simulink model "EstudioVirtual"  (Simulink 7.9)
settings: Solver=ode3  SolverMode=SingleTasking  StartTime=0.0  StopTime=10.0  RelTol=1e-3
PreLoadFcn:
  | waijung.modelPreload; % Required for working with Waijung Blockset. Do not remove.
undefined symbols (not defined in the file or in its folder): ARM, Link, LQFP100, MDK, ST, STM32F407VG, STM32F4DISCOVERY
libraries: stm32f4_io_lib x4, stm32f4_device_config_lib x1
CloseFcn:
  | waijung.modelClose; % Required for working with Waijung Blockset. Do not remove.
settings Model: Creator=Lithium  LastModifiedBy=Lithium
settings OptimizationCC: OptimizeModelRefInitCode=on  LifeSpan=1
settings HardwareCC: ProdEndianess=LittleEndian  ProdHWDeviceType=ARM Compatible->Cortex - M4  TargetEndianess=LittleEndian  TargetHWDeviceType=ARM Compatible->Cortex - M4
settings RTWCC: SystemTargetFile=stm32f4.tlc  GenerateMakefile=off  TemplateMakefile=ert_default_tmf  Description=STM32F4 Target  ProcessScript=stm32f4_make_rtw_hook
settings CodeAppCC: IgnoreCustomStorageClasses=off
settings STFCustomTargetCC: CodeReplacementLibrary=ANSI_C  ModelReferenceCompliant=off  CombineOutputUpdateFcns=on  ERTCustomFileBanners=on  SupportContinuousTime=off  SupportNonInlinedSFcns=off  GRTInterface=off  SystemTargetFile=stm32f4.tlc
settings ERTTargetCC: CodeReplacementLibrary=ANSI_C  MultiwordLength=2048  ModelReferenceCompliant=off  ParMdlRefBuildCompliant=off  CompOptLevelCompliant=off  ConcurrentExecutionCompliant=off  ERTFirstTimeCompliant=off  ModelStepFunctionPrototypeControlCompliant=off  CPPClassGenCompliant=off  InlinedParameterPlacement=NonHierarchical  ERTSrcFileBannerTemplate=stm32f4_code_template.cgt  ERTHdrFileBannerTemplate=stm32f4_code_template.cgt  ERTDataSrcFileTemplate=stm32f4_code_template.cgt  ERTDataHdrFileTemplate=stm32f4_code_template.cgt  ERTCustomFileTemplate=stm32f4_file_process.tlc  ConvertIfToSwitch=off  SuppressUnreachableDefaultCases=off

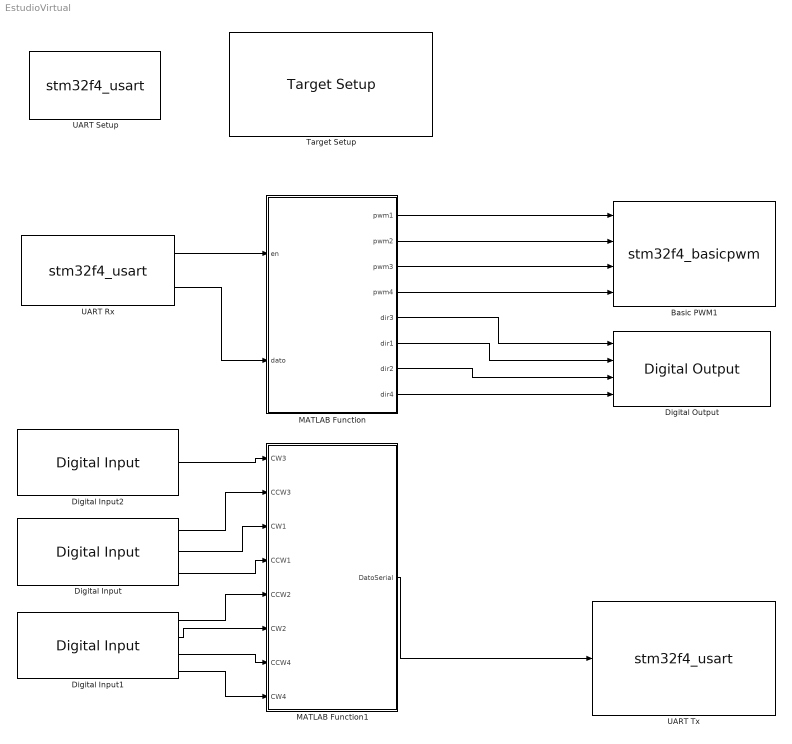
== system EstudioVirtual ==
  Basic PWM1 : S-Function  FunctionName=stm32f4_basicpwm  Parameters=timer,pwmperiod,ch1pin,ch2pin,ch3pin,ch4pin,sampletime,sampletimestr,blockid,apb,portstr,pinstr,pinmat,timarr,timprescale,chmat,polaritystr  EnableBusSupport=off  mask(stm32f4_basicpwm){timer=1, pwmperiod=0.0001, polarity=Active High, polaritystr=TIM_OCPolarity_High, ch1pin=E9, ch2pin=E11, ch3pin=E13, ch4pin=E14, sampletime=0.01, sampletimestr=-1, blockid=BasicPWM1, portpinstr=E9,E11,E13,E14, enablecustomportlabel=on, cinputportlabel=PWM1, PWM2, PWM3, PWM4, coutputportlabel=0, apb=2, portstr=["E"], pinstr=["GPIO_Pin_9 | GPIO_Pin_11 | GPIO_Pin_13 | GPIO_Pin_14"], pinmat=[4 9 11 13 14], timarr=16799, timprescale=0, chmat=[1  2  3  4]}
      mask prompts: pwmperiod "PWM Period (seconds)"; ch1pin "Channel 1"; ch2pin "Channel 2"; ch3pin "Channel 3"; ch4pin "Channel 4"; sampletime "Sample time (sec)"; sampletimestr "Compiled sample time (sec) in string"; portpinstr "Port pin string"; enablecustomportlabel "Enable custom port labels"; cinputportlabel "Custom input port labels (Ex. In1, In2, In3)"; coutputportlabel "Custom output port labels (Ex. Out1, Out2, Out3)"; portstr "Port string"; pinstr "Pin string"; pinmat "Pin matrix"; timarr "Timer ARR"; timprescale "Timer PRESCALE"; chmat "Channel order"
      mask help:
      | This block implements basic Edge-aligned Pulse Width Modulation (PWM) generation.
      | All timers are 16-bit. The PWM period is fixed (per timer).
      mask init:
      | stm32f4_basicpwm_callback('init');
      mask Help: web(fullfile(waijungdocroot,'stm32f4_basicpwm.htm'),'-browser')
      mask StyleString: popup(1|2|3|4|5|8|9|10|11|12|13|14),edit,popup(Active High|Active Low),edit,popup(Not available - Do not use|E9|A8),popup(Not available - Do not use|E11|A9),popup(Not available - Do not use|E13|A10),popup(Not available - Do not use|E14|A11),edit,edit,edit,edit,checkbox,edit,edit,edit,edit,edit,edit,edit,edit,edit
      mask CallbackString: stm32f4_basicpwm_callback('timer');|stm32f4_basicpwm_callback('pwmperiod');|stm32f4_basicpwm_callback('polarity');||stm32f4_basicpwm_callback('ch1pin');|stm32f4_basicpwm_callback('ch2pin');|stm32f4_basicpwm_callback('ch3pin');|stm32f4_basicpwm_callback('ch4pin');|stm32f4_basicpwm_callback('sampletime');|stm32f4_basicpwm_callback('sampletimestr');|stm32f4_basicpwm_callback('blockid');||stm32f4_basicpwm_callback('enablecustomportlabel');|||||||||
      mask Display: text(0.95, 0.5, 'Timer: 1\nPolarity: Active High\nPeriod (sec) 0.0001\nTs (sec): -1','ver','middle','hor','right');port_label('input', 1,'PWM1 (E9)');port_label('input', 2,'PWM2 (E11)');port_label('input', 3,'PWM3 (E13)');port_label('input', 4,'PWM4 (E14)')
  Digital Input : stm32f4_io_lib/Digital Input  port=B  speed=100  porttype=Pull Up  porttypestr=UP  use_pin0=off  use_pin1=off  use_pin2=off  use_pin3=on  use_pin4=off  use_pin5=off  use_pin6=off  use_pin7=off  use_pin8=off  use_pin9=off  use_pin10=off  use_pin11=off  use_pin12=off  use_pin13=on  use_pin14=on  use_pin15=off  pinstr=GPIO_Pin_3 | GPIO_Pin_13 | GPIO_Pin_14  usedpinarray="[0  0  0  1  0  0  0  0  0  0  0  0  0  1  1  0]"  bitbandingstr=|  sampletime=0.01  sampletimestr=-1  blockid=DigitalInput  enablecustomportlabel=on  glabalinit=off  cinputportlabel=In1, In2  coutputportlabel=CCW3, CW1, CCW1
      | #define DigitalInput_B3 Peripheral_BB(GPIOB->IDR, 3)  /* Output pin */
      | #define DigitalInput_B13 Peripheral_BB(GPIOB->IDR, 13)  /* Output pin */
      | #define DigitalInput_B14 Peripheral_BB(GPIOB->IDR, 14)  /* Output pin */
  Digital Input1 : stm32f4_io_lib/Digital Input  port=E  speed=100  porttype=Pull Up  porttypestr=UP  use_pin0=off  use_pin1=off  use_pin2=off  use_pin3=off  use_pin4=off  use_pin5=on  use_pin6=on  use_pin7=on  use_pin8=off  use_pin9=off  use_pin10=off  use_pin11=off  use_pin12=on  use_pin13=off  use_pin14=off  use_pin15=off  pinstr=GPIO_Pin_5 | GPIO_Pin_6 | GPIO_Pin_7 | GPIO_Pin_12  usedpinarray="[0  0  0  0  0  1  1  1  0  0  0  0  1  0  0  0]"  bitbandingstr=|  sampletime=0.01  sampletimestr=-1  blockid=DigitalInput1  enablecustomportlabel=on  glabalinit=off  cinputportlabel=In1, In2  coutputportlabel=CCW2, CW2, CCW4, CW4
      | #define DigitalInput1_E5 Peripheral_BB(GPIOE->IDR, 5)  /* Output pin */
      | #define DigitalInput1_E6 Peripheral_BB(GPIOE->IDR, 6)  /* Output pin */
      | #define DigitalInput1_E7 Peripheral_BB(GPIOE->IDR, 7)  /* Output pin */
      | #define DigitalInput1_E12 Peripheral_BB(GPIOE->IDR, 12)  /* Output pin */
  Digital Input2 : stm32f4_io_lib/Digital Input  port=D  speed=100  porttype=Pull Up  porttypestr=UP  use_pin0=off  use_pin1=off  use_pin2=off  use_pin3=off  use_pin4=off  use_pin5=off  use_pin6=off  use_pin7=off  use_pin8=off  use_pin9=off  use_pin10=off  use_pin11=on  use_pin12=off  use_pin13=off  use_pin14=off  use_pin15=off  pinstr=GPIO_Pin_11  usedpinarray="[0  0  0  0  0  0  0  0  0  0  0  1  0  0  0  0]"  bitbandingstr="#define DigitalInput2_D11 Peripheral_BB(GPIOD->IDR, 11)  /* Output pin */"  sampletime=0.01  sampletimestr=-1  blockid=DigitalInput2  enablecustomportlabel=on  glabalinit=off  cinputportlabel=In1, In2  coutputportlabel=CW3
  Digital Output : stm32f4_io_lib/Digital Output  use_bitband=on  port=B  speed=100  porttype=Push Pull  porttypestr=PP  use_pin0=off  use_pin1=off  use_pin2=off  use_pin3=off  use_pin4=on  use_pin5=off  use_pin6=off  use_pin7=on  use_pin8=on  use_pin9=on  use_pin10=off  use_pin11=off  use_pin12=off  use_pin13=off  use_pin14=off  use_pin15=off  pinstr=GPIO_Pin_4 | GPIO_Pin_7 | GPIO_Pin_8 | GPIO_Pin_9  usedpinarray="[0  0  0  0  1  0  0  1  1  1  0  0  0  0  0  0]"  bitbandingstr=|  sampletime=-1  sampletimestr=-1  blockid=DigitalOutput  enablecustomportlabel=on  globalinit=off  cinputportlabel=Dir3, Dir1, Dir2, Dir4  coutputportlabel=0
      | #define DigitalOutput_B4 Peripheral_BB(GPIOB->ODR, 4)  /* Output pin */
      | #define DigitalOutput_B7 Peripheral_BB(GPIOB->ODR, 7)  /* Output pin */
      | #define DigitalOutput_B8 Peripheral_BB(GPIOB->ODR, 8)  /* Output pin */
      | #define DigitalOutput_B9 Peripheral_BB(GPIOB->ODR, 9)  /* Output pin */
  MATLAB Function : MATLAB Function  TreatAsAtomicUnit=on
  MATLAB Function1 : MATLAB Function  TreatAsAtomicUnit=on
  Target Setup : stm32f4_device_config_lib/Target Setup  Priority=100  compiler=MDK-ARM  previous_compiler=MDK-ARM  mcu=STM32F407VG (LQFP100); STM32F4DISCOVERY  mcustr=STM32F407VG  clockconfig=STM32F4DISCOVERY Default (HSEOSC-8MHz/HCLK-168MHz)  system_stm32f4xx_c_path=C:\Users\Lithium\Downloads\waijung14_12a\targets\stm32f4_target\stm32f4\utils\STM32F4xx_AN3988_V1.0.1\stm32f4_default\hseosc8mhz  showmemoryconfiguration=off  stacksize=0x2000  heapsize=0x2000  enableautocompiledownload=on  fullchiperase=off  programmerinterface=ST-Link  editctrlstr=on  compilercontrolstr=-c --cpu Cortex-M4.fp -g -O3 --apcs=interwork --split_sections $(INCLUDES)  assemblercontrolstr="--cpu Cortex-M4.fp -g --apcs=interwork  --xref $(INCLUDES)"  linkercontrolstr="--cpu Cortex-M4.fp --strict --scatter \"$(MODELNAME).sct\" --summary_stderr --info summarysizes --map --xref --callgraph --symbols --info sizes --info totals --info unused --info veneers  --list \".\\$(MODELNAME).map\" -o $(MODELNAME).axf"  runafterdownload=on  execprofile=None  profileruart=3  profilerbaud=500000  profilertxpin=D8  profilerinitstr=0.01,168000000,1680000,500000,0  manualsetsampletime=off  sampletime=0.01  blockid=TargetSetup  systickreloadvalue=1680000  hseval=8000000  lastprofileruart=3  hclk=168000000  flashorigin=0x08000000  flashlength=0x00100000  ramorigin=0x20000000  ramlength=0x00020000  useextram=off
  UART Rx : S-Function  Priority=1  FunctionName=stm32f4_usart  Parameters=configuration,uartmodule,transfer,baudrate,inputtype,outputtype,confstr,binheaderarray,binterminatorarray,asciiheader,asciiterminator,bindatalength,packetmode,varname,sampletime,sampletimestr,blockid  EnableBusSupport=off  mask(stm32f4_usart){configuration=Rx, uartmodule=6, baudrate=115200, databits=8, parity=No, stopbit=1, remaptxpin=Not used, remaprxpin=Not used, flowcontrol=None, remapctspin=Not used, remaprtspin=Not used, advanceoptions=off, rxbuffersize=512, txbuffersize=512, transfer=Non-Blocking, packetmode=Binary Vector, binheader='S', binterminator='0E', porttype_double=0, porttype_single=0, porttype_int8=3, porttype_uint8=0, porttype_int16=0, porttype_uint16=0, porttype_int32=0, porttype_uint32=0, asciiformat='value=%d,%f', rx_asciiterminator=CRLF (0x0D 0x0A - "\\r\\n"), tx_asciiterminator=LF (0x0A - "\\n"), storagename=<empty>, varname=, inputtype=[0], outputtype=[2 3  770], binheaderarray=[2 126  126], binterminatorarray=[1 14], bindatalength=3, asciiheader='value=%d,%f\\r\\n', asciiterminator=[2 13 10], sampletime=-1, sampletimestr=-1, blockid=UARTRx, confstr=[ "dummy", "0", "*", "*", "0", "*", "*", "0", "*", "*", "0", "*", "*", "2", "5", "6", "2", "5", "1", "512", "512", "2", "6", "115200", "8", "No", "1", "None", "USART6"], lastmodule=1}
      mask prompts: uartmodule "UART Module"; baudrate "Baud rate (bps)"; databits "Data bits"; stopbit "Stop bit"; remaptxpin "Tx Pin"; remaprxpin "Rx Pin"; flowcontrol "Hardware flow control"; remapctspin "HW Flow control, CTS Pin"; remaprtspin "HW Flow control, RTS Pin"; advanceoptions "Advance options"; rxbuffersize "Rx buffer size (bytes)"; txbuffersize "Tx buffer size (bytes)"; packetmode "Packet mode"; binheader "Binary header (example: '7E 7E')"; binterminator "Binary terminator (example: '03 03')"; porttype_double "Number of data port, type DOUBLE"; porttype_single "Number of data port, type SINGLE"; porttype_int8 "Number of data port, type INT8"; porttype_uint8 "Number of data port, type UINT8"; porttype_int16 "Number of data port, type INT16"; porttype_uint16 "Number of data port, type UINT16"; porttype_int32 "Number of data port, type INT32"; porttype_uint32 "Number of data port, type UINT32"; asciiformat "Ascii format"; rx_asciiterminator "End of packet"; tx_asciiterminator "End of packet"; storagename "Buffer"; varname "Var name"; inputtype "Input data type"; outputtype "Output data type"; binheaderarray "Binary header"; binterminatorarray "Binary terminator"; bindatalength "Binary data length"; asciiheader "Ascii header (printf format)"; asciiterminator "Ascii terminator"; sampletime "Sample time (sec)"; sampletimestr "Compiled sample time (sec) in string"; confstr "Configuration string"; lastmodule "Last module selected"
      mask help:
      | Data type for Ascii format
      | %u, %i, %d, %o, %x: uint32
      | %e, %g, %f: single
      | %c: int8
      mask init:
      | stm32f4_usart_callback('init');
      mask Help: web(fullfile(waijungdocroot,'stm32f4_usart_rx.htm'), '-browser')
      mask StyleString: popup(Setup|Tx|Rx),popup(1|2|3|4|5|6),edit,popup(8),popup(No|Odd|Even),popup(0.5|1|1.5|2),popup(Not used|A9|B6),popup(Not used|A10|B7),popup(None|RTS|CTS|RTS/CTS),popup(Not used|A11),popup(Not used|A12),checkbox,popup(16|32|64|128|256|512|1024|2048),popup(16|32|64|128|256|512|1024|2048),popup(Blocking|Non-Blocking),popup(Ascii|Binary|Binary Vector|String Buffer),edit,edit,edit,edit,edit,edit,edit,edit,edit,edit,edit,popup(CR (0x0D - "\\\\r")|LF (0x0A - "\\\\n")|CRLF (0x0D 0x0A - "\\\\r\\\\n")),popup(CR (0x0D - "\\\\r")|LF (0x0A - "\\\\n")|CRLF (0x0D 0x0A - "\\\\r\\\\n")|None),popup(<empty>),edit,edit,edit,edit,edit,edit,edit,edit,edit,edit,edit,edit,edit
      mask CallbackString: stm32f4_usart_callback('configuration');|stm32f4_usart_callback('uartmodule');|stm32f4_usart_callback('baudrate');||||||stm32f4_usart_callback('flowcontrol');|||stm32f4_usart_callback('advanceoptions');|||stm32f4_usart_callback('transfer');|stm32f4_usart_callback('packetmode');|stm32f4_usart_callback('binheader');|stm32f4_usart_callback('binterminator');|stm32f4_usart_callback('porttype');|stm32f4_usart_callback('porttype');|stm32f4_usart_callback('porttype');|stm32f4_usart_callback('porttype');|stm32f4_usart_callback('porttype');|stm32f4_usart_callback('porttype');|stm32f4_usart_callback('porttype');|stm32f4_usart_callback('porttype');|stm32f4_usart_callback('asciiformat');|stm32f4_usart_callback('rx_asciiterminator');|stm32f4_usart_callback('tx_asciiterminator');|stm32f4_usart_callback('storagename');|stm32f4_usart_callback('varname');||||||||stm32f4_usart_callback('sampletime');|stm32f4_usart_callback('sampletimestr');|stm32f4_usart_callback('blockid');||
      mask Display: text(0.05, 0.5, 'Module: USART6_Rx\nPacket: Binary Vector\nTransfer: Non-Blocking\nTs (sec): -1','ver','middle','hor','left'); port_label('output', 1,'READY'); port_label('output', 2,'int8(3)');
  UART Setup : S-Function  Priority=1  FunctionName=stm32f4_usart  Parameters=configuration,uartmodule,transfer,baudrate,inputtype,outputtype,confstr,binheaderarray,binterminatorarray,asciiheader,asciiterminator,bindatalength,packetmode,varname,sampletime,sampletimestr,blockid  EnableBusSupport=off  mask(stm32f4_usart){configuration=Setup, uartmodule=6, baudrate=9600, databits=8, parity=No, stopbit=1, remaptxpin=C6, remaprxpin=C7, flowcontrol=None, remapctspin=Not used, remaprtspin=Not used, advanceoptions=off, rxbuffersize=512, txbuffersize=512, transfer=Blocking, packetmode=Ascii, binheader='7E 7E', binterminator='03 03', porttype_double=1, porttype_single=0, porttype_int8=1, porttype_uint8=0, porttype_int16=0, porttype_uint16=0, porttype_int32=0, porttype_uint32=0, asciiformat='%d,%f', rx_asciiterminator=CRLF (0x0D 0x0A - "\\r\\n"), tx_asciiterminator=CR (0x0D - "\\r"), storagename=<empty>, varname=, inputtype=[0], outputtype=[0], binheaderarray=[0], binterminatorarray=[0], bindatalength=0, asciiheader='', asciiterminator=[0], sampletime=-1, sampletimestr=-1, blockid=UARTSetup, confstr=[ "dummy", "1", "C", "6", "1", "C", "7", "0", "*", "*", "0", "*", "*", "2", "5", "6", "2", "5", "1", "512", "512", "2", "6", "9600", "8", "No", "1", "None", "USART6"], lastmodule=6}
      mask prompts: uartmodule "UART Module"; baudrate "Baud rate (bps)"; databits "Data bits"; stopbit "Stop bit"; remaptxpin "Tx Pin"; remaprxpin "Rx Pin"; flowcontrol "Hardware flow control"; remapctspin "HW Flow control, CTS Pin"; remaprtspin "HW Flow control, RTS Pin"; advanceoptions "Advance options"; rxbuffersize "Rx buffer size (bytes)"; txbuffersize "Tx buffer size (bytes)"; packetmode "Packet mode"; binheader "Binary header (example: '7E 7E')"; binterminator "Binary terminator (example: '03 03')"; porttype_double "Number of data port, type DOUBLE"; porttype_single "Number of data port, type SINGLE"; porttype_int8 "Number of data port, type INT8"; porttype_uint8 "Number of data port, type UINT8"; porttype_int16 "Number of data port, type INT16"; porttype_uint16 "Number of data port, type UINT16"; porttype_int32 "Number of data port, type INT32"; porttype_uint32 "Number of data port, type UINT32"; asciiformat "Ascii format"; rx_asciiterminator "End of packet"; tx_asciiterminator "End of packet"; storagename "Buffer"; varname "Var name"; inputtype "Input data type"; outputtype "Output data type"; binheaderarray "Binary header"; binterminatorarray "Binary terminator"; bindatalength "Binary data length"; asciiheader "Ascii header (printf format)"; asciiterminator "Ascii terminator"; sampletime "Sample time (sec)"; sampletimestr "Compiled sample time (sec) in string"; confstr "Configuration string"; lastmodule "Last module selected"
      mask help:
      | Default STM32F4DISCOVERY + aMG F4 Connect 2 + aMG USB Converter N2 settings use
      |
      | USART3, Tx D8, Rx D9 and USB Serial Converter A.
      mask init:
      | stm32f4_usart_callback('init');
      mask Help: web(fullfile(waijungdocroot,'stm32f4_usart_setup.htm'), '-browser')
      mask StyleString: popup(Setup|Tx|Rx),popup(1|2|3|4|5|6),edit,popup(8),popup(No|Odd|Even),popup(0.5|1|1.5|2),popup(Not used|C6),popup(Not used|C7),popup(None|RTS|CTS|RTS/CTS),popup(Not used),popup(Not used),checkbox,popup(16|32|64|128|256|512|1024|2048),popup(16|32|64|128|256|512|1024|2048),popup(Blocking|Non-Blocking),popup(Ascii|Binary|String Buffer),edit,edit,edit,edit,edit,edit,edit,edit,edit,edit,edit,popup(CR (0x0D - "\\\\r")|LF (0x0A - "\\\\n")|CRLF (0x0D 0x0A - "\\\\r\\\\n")),popup(CR (0x0D - "\\\\r")|LF (0x0A - "\\\\n")|CRLF (0x0D 0x0A - "\\\\r\\\\n")|None),popup(<empty>),edit,edit,edit,edit,edit,edit,edit,edit,edit,edit,edit,edit,edit
      mask CallbackString: stm32f4_usart_callback('configuration');|stm32f4_usart_callback('uartmodule');|stm32f4_usart_callback('baudrate');||||||stm32f4_usart_callback('flowcontrol');|||stm32f4_usart_callback('advanceoptions');|||stm32f4_usart_callback('transfer');|stm32f4_usart_callback('packetmode');|stm32f4_usart_callback('binheader');|stm32f4_usart_callback('binterminator');|stm32f4_usart_callback('porttype');|stm32f4_usart_callback('porttype');|stm32f4_usart_callback('porttype');|stm32f4_usart_callback('porttype');|stm32f4_usart_callback('porttype');|stm32f4_usart_callback('porttype');|stm32f4_usart_callback('porttype');|stm32f4_usart_callback('porttype');|stm32f4_usart_callback('asciiformat');|stm32f4_usart_callback('rx_asciiterminator');|stm32f4_usart_callback('tx_asciiterminator');|stm32f4_usart_callback('storagename');|stm32f4_usart_callback('varname');||||||||stm32f4_usart_callback('sampletime');|stm32f4_usart_callback('sampletimestr');|stm32f4_usart_callback('blockid');||
      mask Display: text(0.5, 0.5, 'Module: USART6_Setup\nBaud (Bps): 9600\nDMA Buffer: 512/512\nTx/Rx Pin: C6/C7','ver','middle','hor','center');
  UART Tx : S-Function  Priority=1  FunctionName=stm32f4_usart  Parameters=configuration,uartmodule,transfer,baudrate,inputtype,outputtype,confstr,binheaderarray,binterminatorarray,asciiheader,asciiterminator,bindatalength,packetmode,varname,sampletime,sampletimestr,blockid  EnableBusSupport=off  mask(stm32f4_usart){configuration=Tx, uartmodule=6, baudrate=115200, databits=8, parity=No, stopbit=1, remaptxpin=Not used, remaprxpin=Not used, flowcontrol=None, remapctspin=Not used, remaprtspin=Not used, advanceoptions=off, rxbuffersize=512, txbuffersize=512, transfer=Non-Blocking, packetmode=Binary Vector, binheader='S', binterminator='0E', porttype_double=0, porttype_single=0, porttype_int8=4, porttype_uint8=0, porttype_int16=0, porttype_uint16=0, porttype_int32=0, porttype_uint32=0, asciiformat='value=%d,%f', rx_asciiterminator=CRLF (0x0D 0x0A - "\\r\\n"), tx_asciiterminator=CRLF (0x0D 0x0A - "\\r\\n"), storagename=<empty>, varname=, inputtype=[1  1026], outputtype=[0], binheaderarray=[1 14], binterminatorarray=[1 14], bindatalength=4, asciiheader='value=%d,%f\\r\\n', asciiterminator=[2 13 10], sampletime=-1, sampletimestr=-1, blockid=UARTTx, confstr=[ "dummy", "0", "*", "*", "0", "*", "*", "0", "*", "*", "0", "*", "*", "2", "5", "6", "2", "5", "1", "512", "512", "2", "6", "115200", "8", "No", "1", "None", "USART6"], lastmodule=1}
      mask prompts: uartmodule "UART Module"; baudrate "Baud rate (bps)"; databits "Data bits"; stopbit "Stop bit"; remaptxpin "Tx Pin"; remaprxpin "Rx Pin"; flowcontrol "Hardware flow control"; remapctspin "HW Flow control, CTS Pin"; remaprtspin "HW Flow control, RTS Pin"; advanceoptions "Advance options"; rxbuffersize "Rx buffer size (bytes)"; txbuffersize "Tx buffer size (bytes)"; packetmode "Packet mode"; binheader "Binary header (example: '7E 7E')"; binterminator "Binary terminator (example: '03 03')"; porttype_double "Number of data port, type DOUBLE"; porttype_single "Number of data port, type SINGLE"; porttype_int8 "Number of data port, type INT8"; porttype_uint8 "Number of data port, type UINT8"; porttype_int16 "Number of data port, type INT16"; porttype_uint16 "Number of data port, type UINT16"; porttype_int32 "Number of data port, type INT32"; porttype_uint32 "Number of data port, type UINT32"; asciiformat "Ascii format"; rx_asciiterminator "End of packet"; tx_asciiterminator "End of packet"; storagename "Buffer"; varname "Var name"; inputtype "Input data type"; outputtype "Output data type"; binheaderarray "Binary header"; binterminatorarray "Binary terminator"; bindatalength "Binary data length"; asciiheader "Ascii header (printf format)"; asciiterminator "Ascii terminator"; sampletime "Sample time (sec)"; sampletimestr "Compiled sample time (sec) in string"; confstr "Configuration string"; lastmodule "Last module selected"
      mask help:
      | Data type for Ascii format
      | %u, %i, %d, %o, %x: uint32
      | %e, %g, %f: single
      | %c: int8
      mask init:
      | stm32f4_usart_callback('init');
      mask Help: web(fullfile(waijungdocroot,'stm32f4_usart_tx.htm'), '-browser')
      mask StyleString: popup(Setup|Tx|Rx),popup(1|2|3|4|5|6),edit,popup(8),popup(No|Odd|Even),popup(0.5|1|1.5|2),popup(Not used|A9|B6),popup(Not used|A10|B7),popup(None|RTS|CTS|RTS/CTS),popup(Not used|A11),popup(Not used|A12),checkbox,popup(16|32|64|128|256|512|1024|2048),popup(16|32|64|128|256|512|1024|2048),popup(Blocking|Non-Blocking),popup(Ascii|Binary|Binary Vector|String Buffer),edit,edit,edit,edit,edit,edit,edit,edit,edit,edit,edit,popup(CR (0x0D - "\\\\r")|LF (0x0A - "\\\\n")|CRLF (0x0D 0x0A - "\\\\r\\\\n")),popup(CR (0x0D - "\\\\r")|LF (0x0A - "\\\\n")|CRLF (0x0D 0x0A - "\\\\r\\\\n")|None),popup(<empty>),edit,edit,edit,edit,edit,edit,edit,edit,edit,edit,edit,edit,edit
      mask CallbackString: stm32f4_usart_callback('configuration');|stm32f4_usart_callback('uartmodule');|stm32f4_usart_callback('baudrate');||||||stm32f4_usart_callback('flowcontrol');|||stm32f4_usart_callback('advanceoptions');|||stm32f4_usart_callback('transfer');|stm32f4_usart_callback('packetmode');|stm32f4_usart_callback('binheader');|stm32f4_usart_callback('binterminator');|stm32f4_usart_callback('porttype');|stm32f4_usart_callback('porttype');|stm32f4_usart_callback('porttype');|stm32f4_usart_callback('porttype');|stm32f4_usart_callback('porttype');|stm32f4_usart_callback('porttype');|stm32f4_usart_callback('porttype');|stm32f4_usart_callback('porttype');|stm32f4_usart_callback('asciiformat');|stm32f4_usart_callback('rx_asciiterminator');|stm32f4_usart_callback('tx_asciiterminator');|stm32f4_usart_callback('storagename');|stm32f4_usart_callback('varname');||||||||stm32f4_usart_callback('sampletime');|stm32f4_usart_callback('sampletimestr');|stm32f4_usart_callback('blockid');||
      mask Display: text(0.5, 0.5, 'Module: USART6_Tx\nPacket: Binary Vector\nTransfer: Non-Blocking\nTs (sec): -1','ver','middle','hor','center'); port_label('input', 1,'int8(4)');
  wires:
  UART Rx/1 -> MATLAB Function/1(en)
  UART Rx/2 -> MATLAB Function/2(dato)
  MATLAB Function/2(pwm2) -> Basic PWM1/2
  MATLAB Function/3(pwm3) -> Basic PWM1/3
  MATLAB Function/4(pwm4) -> Basic PWM1/4
  MATLAB Function/1(pwm1) -> Basic PWM1/1
  MATLAB Function/5(dir3) -> Digital Output/1
  MATLAB Function/6(dir1) -> Digital Output/2
  MATLAB Function/8(dir4) -> Digital Output/4
  MATLAB Function/7(dir2) -> Digital Output/3
  Digital Input2/1 -> MATLAB Function1/1(CW3)
  Digital Input/1 -> MATLAB Function1/2(CCW3)
  Digital Input/2 -> MATLAB Function1/3(CW1)
  Digital Input/3 -> MATLAB Function1/4(CCW1)
  Digital Input1/1 -> MATLAB Function1/5(CCW2)
  Digital Input1/2 -> MATLAB Function1/6(CW2)
  Digital Input1/3 -> MATLAB Function1/7(CCW4)
  Digital Input1/4 -> MATLAB Function1/8(CW4)
  MATLAB Function1/1(DatoSerial) -> UART Tx/1

== matlab function MATLAB Function1 ==
  data: CW3 input double; CCW3 input double; CW1 input double; CCW1 input double; CCW2 input double; CW2 input double; CCW4 input double; CW4 input double; DatoSerial output double
function DatoSerial  = fcn(CW3, CCW3, CW1, CCW1, CCW2, CW2, CCW4, CW4)
%#codegen

contador1 = int16(0);
Posicion1 = int16(0);
contador2 = int16(0);
Posicion2 = int16(0);
contador3 = int16(0);
Posicion3 = int16(0);
contador4 = int16(0);
Posicion4 = int16(0);
DatoSerial = [0, 0, 0, 0, 0, 0];

%Encoder 1
if (CW1 == 1)
    contador1 = contador1 + 1;
end

if (CCW1 == 1)
    contador1 = contador1 - 1;
end

%Encoder 2
if (CW2 == 1)
    contador2 = contador2 + 1;
end

if (CCW2 == 1)
    contador2 = contador2 - 1;
end

%Encoder 3
if (CW3 == 1)
    contador3 = contador3 + 1;
end

if (CCW3 == 1)
    contador3 = contador3 - 1;
end

%Encoder 4
if (CW4 == 1)
    contador4 = contador4 + 1;
end

if (CCW4 == 1)
    contador4 = contador4 - 1;
end

%127/180 se empaqueta para ser enviado por el puerto serial
Posicion1 = (360/12000)*contador1*(127/180);
Posicion2 = (360/15000)*contador1*(127/180);
Posicion3 = (360/30000)*contador1*(127/180);
Posicion4 = (360/3150)*contador1*(127/180);


%Envio de las posiciones por el puerto serial
DatoSerial(1) = 'S';
DatoSerial(2) = Posicion1;
DatoSerial(3) = Posicion2;
DatoSerial(4) = Posicion3;
DatoSerial(5) = Posicion4;
DatoSerial(6) = 'E';

== matlab function MATLAB Function ==
  data: en input double; pwm1 output double; pwm2 output double; pwm3 output double; pwm4 output double; dir3 output double; dato input double; dir1 output double; dir2 output double; dir4 output double
function [pwm1,pwm2,pwm3,pwm4, dir3, dir1, dir2, dir4]= fcn(en, dato)
%#codegen

pwm1 = uint16(0);
pwm2 = uint16(0);
pwm3 = uint16(0);
pwm4 = uint16(0);


if (en)
 
% Control del motor 1    
  if (dato(2) == '1' & dato(2) ~= '0')
     pwm1 = uint16(50);
     if (dato(3) == '1')
         dir1 = uint16(1);
     else
         dir1 = uint16(0);
     end
  else
      pwm1 = uint16(0);
  end
  
  % Control del motor 2   
  if (dato(2) == '2' & dato(2) ~= '0')
     pwm2 = uint16(50);
     if (dato(3) == '1')
         dir2 = uint16(1);
     else
         dir2 = uint16(0);
     end
  else
      pwm2 = uint16(0);
  end
  
  % Control del motor 3   
  if (dato(2) == '3' & dato(2) ~= '0')
     pwm3 = uint16(50);
     if (dato(3) == '1')
         dir3 = uint16(1);
     else
         dir3 = uint16(0);
     end
  else
      pwm3 = uint16(0);
  end
  
  % Control del motor 4   
  if (dato(2) == '4' & dato(2) ~= '0')
     pwm4 = uint16(50);
     if (dato(3) == '1')
         dir4 = uint16(1);
     else
         dir4 = uint16(0);
     end
  else
      pwm4 = uint16(0);
  end
end
